simulink model "Simm_Q11"  (R2023b)
settings: Solver=VariableStepAuto  StartTime=0.0  StopTime=6  RelTol=1e-3
settings Model: Creator=Lucas  LastModifiedBy=Lucas

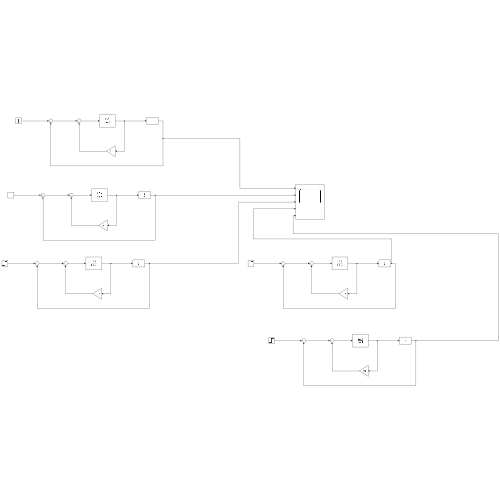
[thumbnail: Simulink's stored preview of the top-level diagram]
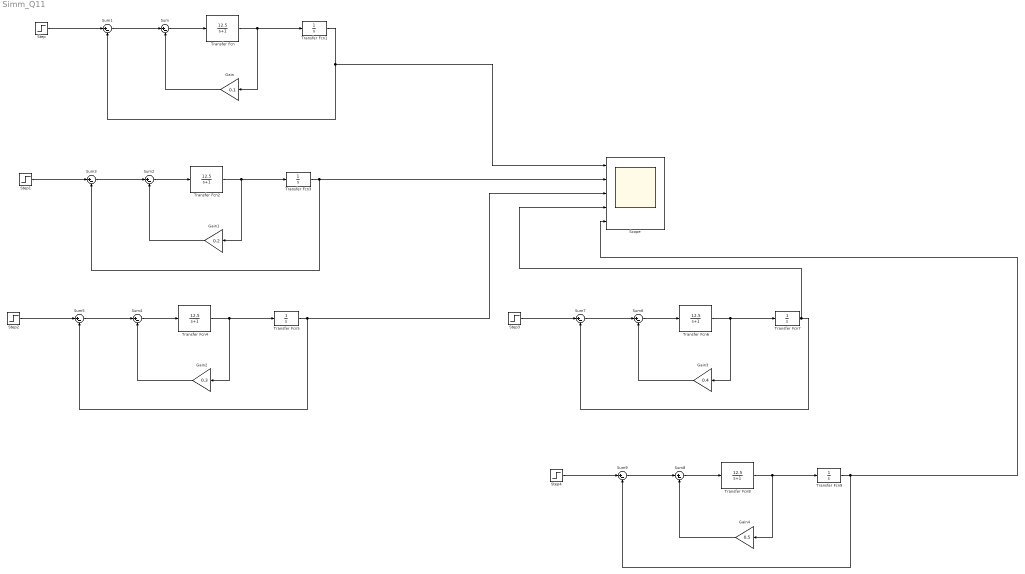
== system Simm_Q11 ==
  Gain : Gain  Gain=0.1
  Gain1 : Gain  Gain=0.2
  Gain2 : Gain  Gain=0.3
  Gain3 : Gain  Gain=0.4
  Gain4 : Gain  Gain=0.5
  Scope : Scope  NumInputPorts=5
  Step{,1..4} (5 alike) : Step  Time=0  SampleTime=0
  Sum{,1..9} (10 alike) : Sum  Inputs=|+-
  Transfer Fcn{,2,4,6,8} (5 alike) : TransferFcn  Numerator=[12.5]  Denominator=[1 1]
  Transfer Fcn{1,3,5,7,9} (5 alike) : TransferFcn  Denominator=[1 0]
  wires:
  Gain/1 -> Sum/2
  Step/1 -> Sum1/1
  Sum/1 -> Transfer Fcn/1
  Transfer Fcn1/1 -> Sum1/2, Scope/1
  Sum1/1 -> Sum/1
  Transfer Fcn/1 -> Gain/1, Transfer Fcn1/1
  Gain1/1 -> Sum2/2
  Step1/1 -> Sum3/1
  Sum2/1 -> Transfer Fcn2/1
  Transfer Fcn3/1 -> Scope/2, Sum3/2
  Sum3/1 -> Sum2/1
  Transfer Fcn2/1 -> Gain1/1, Transfer Fcn3/1
  Transfer Fcn5/1 -> Scope/3, Sum5/2
  Sum4/1 -> Transfer Fcn4/1
  Sum5/1 -> Sum4/1
  Transfer Fcn4/1 -> Gain2/1, Transfer Fcn5/1
  Gain2/1 -> Sum4/2
  Step2/1 -> Sum5/1
  Transfer Fcn7/1 -> Scope/4, Sum7/2
  Sum6/1 -> Transfer Fcn6/1
  Sum7/1 -> Sum6/1
  Transfer Fcn6/1 -> Gain3/1, Transfer Fcn7/1
  Gain3/1 -> Sum6/2
  Step3/1 -> Sum7/1
  Transfer Fcn9/1 -> Sum9/2, Scope/5
  Sum8/1 -> Transfer Fcn8/1
  Sum9/1 -> Sum8/1
  Transfer Fcn8/1 -> Gain4/1, Transfer Fcn9/1
  Gain4/1 -> Sum8/2
  Step4/1 -> Sum9/1
